simulink model "NewModelSimFor5Grades"  (R2024b)
settings: Solver=VariableStepAuto  StartTime=0.0  StopTime=10.0  RelTol=1e-3
undefined symbols (not defined in the file): none, videoinput
libraries: visiontextngfix x1, imaqlib x1, pycoexlib x1
settings Model: Creator=mostafa  LastModifiedBy=mostafa

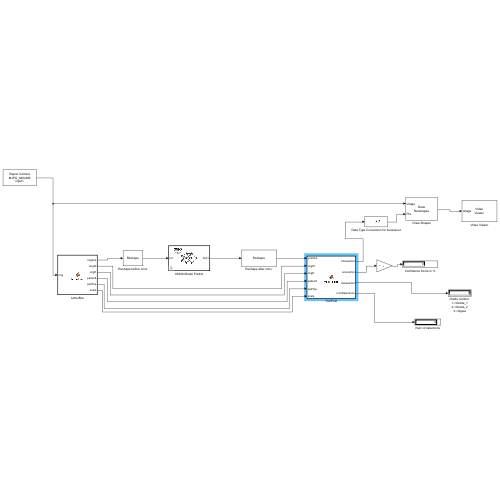
[thumbnail: Simulink's stored preview of the top-level diagram]
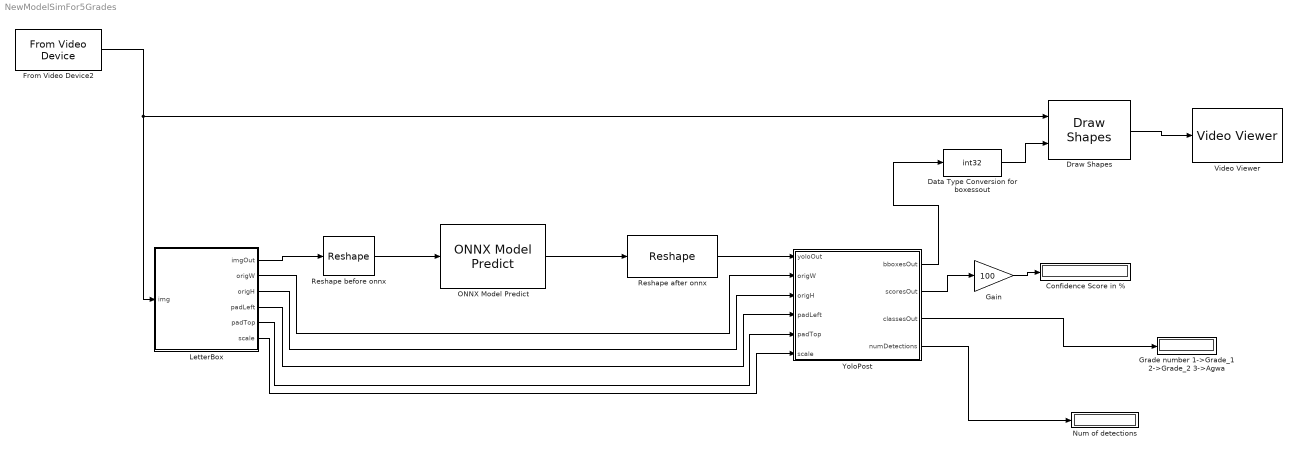
== system NewModelSimFor5Grades ==
  Confidence Score in % : Display
  Data Type Conversion for boxessout : DataTypeConversion  OutDataTypeStr=int32  RndMeth=Nearest  SaturateOnIntegerOverflow=off
  Draw Shapes : visiontextngfix/Draw Shapes  shape=Rectangles  fill=off  lineWidth=1  fillClrSource=Specify via dialog  display=Black  intensity=200  color=[200 255 100]  opacity=0.6  viewport=Entire image  antialiasing=off  inType=Obsolete  imagePorts=One multidimensional signal  roundingMode=Floor  overflowMode=off  memoryMode=Specify word length  memoryWordLength=16  prodOutputMode=Binary point scaling  prodOutputWordLength=32  prodOutputFracLength=14  memoryFracLength=15
  From Video Device2 : imaqlib/From Video Device  DeviceMenu=winvideo 3 (Rapoo Camera)  Device=winvideo 3 (Rapoo Camera)  ObjConstructor=videoinput('winvideo', 3)  VideoFormatMenu=MJPG_640x480  VideoFormat=MJPG_640x480  VideoSource=input1  ROIPosition=[0 0 480 640]  EnableHWTrigger=off  TriggerConfiguration=none/none  SampleTime=1/30  OutputPortsMode=One multidimensional signal  DataType=single  CanDoHWTrigger=no  ReturnedColorSpace=rgb  BlockHandle=435.0006  ROIWidth=640  ROIHeight=480  ROIColumn=0  ROIRow=0  EngXMLPath=C:\Program Files\MATLAB\R2024b\toolbox\imaq\imaq\private  DevXMLPath=C:\ProgramData\MATLAB\SupportPackages\R2024b\toolbox\imaq\supportpackages\genericvideo\adaptor\win64  EngLibPath=C:\Program Files\MATLAB\R2024b\toolbox\imaq\imaqblks\imaqmex\win64  ColorSpace=rgb  BayerSensorAlignment=grbg  ImaqMode=off
  Gain : Gain  Gain=100
  Grade number 1->Grade_1 2->Grade_2 3->Agwa : Display
  LetterBox : MATLAB Function  TreatAsAtomicUnit=on
  Num of detections : Display
  ONNX Model Predict : pycoexlib/ONNX Model Predict  ModelFile=E:\Dates_Project_Final_Run_5Grades\Mejdool_Dates_5Grades\weights\best.onnx  ExecutionProviders=CUDAExecutionProvider, CPUExecutionProvider  InputTable={ 'In1', 'float32', '', '' }  OutputTable={ 'Out1', '', '' }  SampleTime=-1  InputDatatypes=float32  InputPermutations=[]  OutputPermutations=[]  PythonCoexecutionBlockType=ONNXModelBlock  VariableOutputMaxSizes=[]
  "Reshape after onnx " : Reshape  OutputDimensionality=Customize  OutputDimensions=[9 8400]
  Reshape before onnx : Reshape  OutputDimensionality=Customize  OutputDimensions=[1 3 640 640]
  Video Viewer : VideoViewer  FigPos=[545 560.4 417.6 304]
  YoloPost : MATLAB Function  TreatAsAtomicUnit=on
  wires:
  LetterBox/4(padLeft) -> YoloPost/4(padLeft)
  LetterBox/6(scale) -> YoloPost/6(scale)
  YoloPost/2(scoresOut) -> Gain/1
  YoloPost/3(classesOut) -> Grade number 1->Grade_1 2->Grade_2 3->Agwa/1
  Reshape before onnx/1 -> ONNX Model Predict/1
  YoloPost/1(bboxesOut) -> Data Type Conversion for boxessout/1
  LetterBox/2(origW) -> YoloPost/2(origW)
  YoloPost/4(numDetections) -> Num of detections/1
  Gain/1 -> Confidence Score in %/1
  LetterBox/1(imgOut) -> Reshape before onnx/1
  From Video Device2/1 -> LetterBox/1(img), Draw Shapes/1
  LetterBox/3(origH) -> YoloPost/3(origH)
  LetterBox/5(padTop) -> YoloPost/5(padTop)
  Data Type Conversion for boxessout/1 -> Draw Shapes/2
  ONNX Model Predict/1 -> "Reshape after onnx "/1
  "Reshape after onnx "/1 -> YoloPost/1(yoloOut)
  Draw Shapes/1 -> Video Viewer/1

== matlab function NewModelSimFor5Grades/YoloPost ==
  data: yoloOut input single; origW input; origH input; padLeft input; padTop input; scale input; bboxesOut output size=[100 4]; scoresOut output single size=[100 1]; classesOut output single size=[100 1]; numDetections output single size=1
function [bboxesOut, scoresOut, classesOut, numDetections] = yolo_post(yoloOut, origW, origH, padLeft, padTop, scale)
% YOLOv8 Post-Processing (Corrected for 5-Grade Simulink)
    
    % --- 1. Constants ---
    MAX_DETECTIONS = 100;
    CONF_THRESH    = 0.30;
    IOU_THRESH     = 0.45;
    
    % REMOVED: coder.extrinsic causes the mxArray error.
    % selectStrongestBboxMulticlass supports code generation natively.
    % coder.extrinsic('selectStrongestBboxMulticlass'); 
    
    % Initialize Outputs
    bboxesOut     = zeros(MAX_DETECTIONS, 4, 'single');
    scoresOut     = zeros(MAX_DETECTIONS, 1, 'single');
    classesOut    = zeros(MAX_DETECTIONS, 1, 'single');
    numDetections = single(0);
    
    % --- 2. Intelligent Reshaping ---
    % Handle [1x9x8400] or [9x8400]
    rawInput = squeeze(yoloOut);
    [dim1, dim2] = size(rawInput);
    
    % Ensure [8400 x 9] format
    if dim1 < dim2
        raw = rawInput'; 
    else
        raw = rawInput; 
    end
    
    boxesRaw = raw(:, 1:4);       
    classRaw = raw(:, 5:end);     
    
    % --- 3. Filter by Confidence ---
    [maxScores, classIDs] = max(classRaw, [], 2);
    mask = maxScores > CONF_THRESH;
    
    if ~any(mask)
        return; 
    end
    
    b_valid = boxesRaw(mask, :);
    s_valid = maxScores(mask);
    c_valid = classIDs(mask);
    
    % --- 4. Scale Check ---
    % If model outputs normalized (0-1), scale up.
    max_val_check = max(b_valid(:));
    if max_val_check <= 2.0
        b_valid = b_valid * 640.0;
    end
    
    % --- 5. Coordinate Transformation ---
    x = b_valid(:, 1) - b_valid(:, 3) / 2;
    y = b_valid(:, 2) - b_valid(:, 4) / 2;
    w = b_valid(:, 3);
    h = b_valid(:, 4);
    
    % Reverse Letterbox
    x = (x - padLeft) / scale;
    y = (y - padTop) / scale;
    w = w / scale;
    h = h / scale;
    
    % Clip to Image Boundaries
    x = max(0, min(x, origW));
    y = max(0, min(y, origH));
    w = min(w, origW - x);
    h = min(h, origH - y);
    
    valid_area = (w > 1) & (h > 1);
    if ~any(valid_area)
        return;
    end
    
    final_boxes = [x(valid_area) y(valid_area) w(valid_area) h(valid_area)];
    s_valid     = s_valid(valid_area);
    c_valid     = c_valid(valid_area);
    
    % --- 6. NMS (Now runs in Code Gen mode) ---
    [nms_bboxes, nms_scores, nms_classes] = selectStrongestBboxMulticlass( ...
        final_boxes, s_valid, c_valid, ...
        'OverlapThreshold', IOU_THRESH);
        
    % --- 7. Output Assignment ---
    % Define variable size for the intermediate NMS results
    coder.varsize('nms_bboxes', [Inf, 4], [1, 0]);
    coder.varsize('nms_scores', [Inf, 1], [1, 0]);
    coder.varsize('nms_classes', [Inf, 1], [1, 0]);

    if isempty(nms_bboxes)
        return;
    end
    
    count = size(nms_bboxes, 1);
    
    % Robust Min Calculation
    if count > MAX_DETECTIONS
        limit_val = MAX_DETECTIONS;
    else
        limit_val = count;
    end
    
    numDetections = single(limit_val);
    
    % Explicitly cast loop bounds to double
    loop_limit = double(limit_val);
    
    for k = 1:loop_limit
        bboxesOut(k, :)  = nms_bboxes(k, :);
        scoresOut(k, 1)  = nms_scores(k, 1);
        classesOut(k, 1) = nms_classes(k, 1);
    end
end

== matlab function NewModelSimFor5Grades/LetterBox ==
  data: img input; imgOut output single size=[1 3 640 640]; origW output single size=1; origH output single size=1; padLeft output single size=1; padTop output single size=1; scale output single size=1
function [imgOut, origW, origH, padLeft, padTop, scale] = letterbox(img)
% YOLOv8 Pre-processing (Letterbox)
% Uses the "Paste into Canvas" method to avoid padarray errors.

    % --- 1. Output Initialization ---
    % Initialize outputs as single for Simulink ports
    imgOut  = zeros(1, 3, 640, 640, 'single');
    origW   = single(0);
    origH   = single(0);
    padLeft = single(0);
    padTop  = single(0);
    scale   = single(0);

    % Define extrinsic functions
    coder.extrinsic('imresize');

    % --- 2. Setup Constants ---
    TARGET_SIZE = 640; 
    PAD_VALUE   = 114; % Gray value (Standard for YOLO)

    % Get original size
    [h_raw, w_raw, ~] = size(img);
    
    % Assign to output variables
    origH = single(h_raw);
    origW = single(w_raw);

    % --- 3. Calculate Scaling ---
    % Calculate scale factor (keep as double for precision)
    scale_dbl = TARGET_SIZE / max(h_raw, w_raw);
    scale     = single(scale_dbl);

    % Calculate new dimensions
    newW = round(w_raw * scale_dbl);
    newH = round(h_raw * scale_dbl);

    % --- 4. Resize Image ---
    imgResized = imresize(img, [newH newW]);

    % --- 5. Create Canvas & Calculate Offsets ---
    % Create a blank square canvas filled with gray
    % Ensure data types match. If img is uint8, canvas should be uint8.
    if isa(img, 'uint8')
        canvas = repmat(uint8(PAD_VALUE), TARGET_SIZE, TARGET_SIZE, 3);
    else
        canvas = ones(TARGET_SIZE, TARGET_SIZE, 3, 'like', img) * PAD_VALUE;
    end

    % Calculate centering offsets
    padW = TARGET_SIZE - newW;
    padH = TARGET_SIZE - newH;
    
    % Floor division for top/left
    pL = floor(padW / 2);
    pT = floor(padH / 2);
    
    % Assign to outputs
    padLeft = single(pL);
    padTop  = single(pT);

    % --- 6. Paste Image into Canvas ---
    % Calculate start and end indices (1-based for MATLAB)
    rStart = pT + 1;
    rEnd   = pT + newH;
    cStart = pL + 1;
    cEnd   = pL + newW;
    
    % Insert the resized image into the gray canvas
    canvas(rStart:rEnd, cStart:cEnd, :) = imgResized;

    % --- 7. Final Conversion & Normalization ---
    % Convert to single
    imgFloat = single(canvas);
    
    % Normalize to 0-1 (YOLO standard)
    imgFloat = imgFloat / 255.0; 
    
    % Permute: [H, W, C] -> [C, H, W]
    % This is the shape PyTorch/ONNX expects (Planar)
    imgPermuted = permute(imgFloat, [3 1 2]);
    
    % Reshape and Assign to Output Buffer
    imgOut(1, :, :, :) = reshape(imgPermuted, [1, 3, 640, 640]);

end
